simulink model "PathNavShortestRoute"  (R2021a)
settings: Solver=FixedStepDiscrete  StartTime=0.0  StopTime=80  FixedStep=0.01  RelTol=1e-3
values from neighbouring files (symbols this model uses):
  axleLength = 0.136    [robotParameters.m]
  final = makeShort(noZeros)    [createShortPath.m]
  ticksPerRot = 20    [robotParameters.m]
  wheelR = 0.031    [robotParameters.m]
  x = 0.16521    [robotParameters.m]
  y = 0.091117    [robotParameters.m]
undefined symbols (not defined in the file or in its folder): DiscIntNeverNeededParam, InputPWM, lineLength, mapForSim, WheelSpeed
libraries: mobileRoboticsTrainingLib x5, pid_lib x4, simulink_extras x1
settings Model: NumberOfSteps=10  SnapshotBufferSize=100  SnapshotInterval=1  EnablePacing=on  PacingRate=2  Creator=Boitumelo  LastModifiedBy=Marc

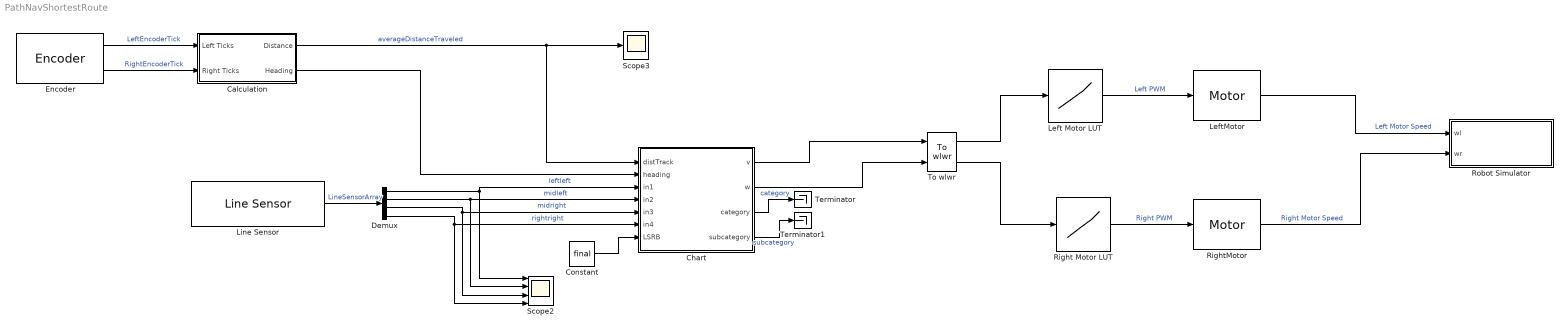
== system PathNavShortestRoute ==
  Calculation : Subsystem
  Chart : Stateflow chart  TreatAsAtomicUnit=on
  Constant : Constant  Value=final
  Demux : Demux
  Encoder : mobileRoboticsTrainingLib/Encoder  axleLength=axleLength  wheelR=wheelR  ticksPerRot=ticksPerRot
      settings: SourceProductName=Mobile Robotics Training Library
  Left Motor LUT : Lookup_n-D  NumberOfTableDimensions=1  BreakpointsForDimension1=WheelSpeed  Table=InputPWM  InterpMethod=Nearest  ExtrapMethod=Clip  InternalRulePriority=Speed  RndMeth=Simplest  InputSameDT=on
  LeftMotor : mobileRoboticsTrainingLib/Motor  motorPlant=wheelMotorModel  sensorType=Speed
      settings: SourceProductName=Mobile Robotics Training Library
  Line Sensor : mobileRoboticsTrainingLib/Line Sensor  mapVariable=mapForSim  envVal=1  lineVal=0  sensOff=[0.0643 0.0354; 0.0675 0.005; 0.0675 -0.005; 0.0643 -0.0354]
      settings: SourceProductName=Mobile Robotics Training Library
  Right Motor LUT : Lookup_n-D  NumberOfTableDimensions=1  BreakpointsForDimension1=WheelSpeed  Table=InputPWM  InterpMethod=Nearest  ExtrapMethod=Clip  InternalRulePriority=Speed  RndMeth=Simplest  InputSameDT=on
  RightMotor : mobileRoboticsTrainingLib/Motor  motorPlant=wheelMotorModel  sensorType=Speed
      settings: SourceProductName=Mobile Robotics Training Library
  Robot Simulator : Subsystem  Priority=99  AncestorBlock=mobileRoboticsTrainingLib/Robot Simulator  mask(Robot Simulator){mapVar=mapForSim, startX=x, startY=y, startTheta=0, axleLength=axleLength, wheelR=wheelR}
      mask prompts: mapVar "Map Variable"; startX "Start X (m)"; startY "Start Y (m)"; startTheta "Theta (deg)"; axleLength "Axle Length (m)"; wheelR "Wheel Radius (m)"
      mask help: Configure robot simulator to use custom simulation maps and simulate closed-loop mobile robotics systems along with appropriate sensor simulation blocks.
      mask init:
      | set_param(bdroot,'SolverType','Fixed-Step');
      | set_param(bdroot,'Solver','FixedStepDiscrete');
      | 
      | if (exist('Ts'))
      |     set_param(bdroot,'FixedStep','Ts');
      | else
      |     set_param(bdroot,'FixedStep','0.01');
      | end
      | 
      | h = findobj('Name','Robot Simulator');
      | if ~isempty(h)
      |     close (h);
      | end
      | setupRobotSim();
      mask Help: web('Robot Simulator.htm')
      mask DialogControl mapCont Prompt: Map Setup
      mask DialogControl initPosCont Prompt: Initial Position
      mask DialogControl setPos Prompt: Set position interactively
      mask DialogControl setPos Callback:
      | %% Set starting point
      | setStartingPoint();
      mask DialogControl initOrientation Prompt: Initial Orientation
      mask DialogControl robotCharCont Prompt: Robot Characteristics
      mask Display: disp('Robot Simulator')
  Scope2 : Scope  NumInputPorts=4
  Scope3 : Scope
  Terminator : Terminator
  Terminator1 : Terminator
  To wlwr : mobileRoboticsTrainingLib/To wlwr  axleLength=0.1  wheelR=0.05
  wires:
  LeftMotor/1 -> Robot Simulator/1(wl)  "Left Motor Speed"
  RightMotor/1 -> Robot Simulator/2(wr)  "Right Motor Speed"
  Right Motor LUT/1 -> RightMotor/1  "Right PWM"
  Left Motor LUT/1 -> LeftMotor/1  "Left PWM"
  To wlwr/1 -> Left Motor LUT/1
  To wlwr/2 -> Right Motor LUT/1
  Line Sensor/1 -> Demux/1  "LineSensorArray"
  Calculation/1(Distance) -> Chart/1(distTrack), Scope3/1  "averageDistanceTraveled"
  Demux/1 -> Scope2/1, Chart/3(in1)  "leftleft"
  Demux/2 -> Scope2/2, Chart/4(in2)  "midleft"
  Demux/3 -> Scope2/3, Chart/5(in3)  "midright"
  Demux/4 -> Scope2/4, Chart/6(in4)  "rightright"
  Chart/1(v) -> To wlwr/1
  Chart/2(w) -> To wlwr/2
  Encoder/1 -> Calculation/1(Left Ticks)  "LeftEncoderTick"
  Encoder/2 -> Calculation/2(Right Ticks)  "RightEncoderTick"
  Calculation/2(Heading) -> Chart/2(heading)
  Chart/3(category) -> Terminator/1  "category"
  Chart/4(subcategory) -> Terminator1/1  "subcategory"
  Constant/1 -> Chart/7(LSRB)

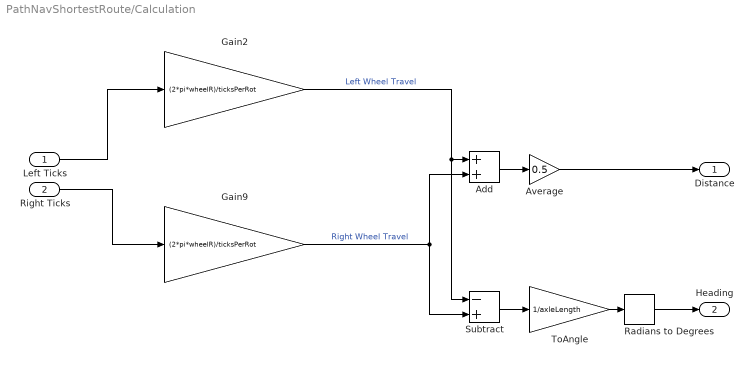
== system PathNavShortestRoute/Calculation ==
  Left Ticks : Inport
  Right Ticks : Inport  Port=2
  Add : Sum
  Average : Gain  Gain=0.5
  Gain2 : Gain  Gain=(2*pi*wheelR)/ticksPerRot
  Gain9 : Gain  Gain=(2*pi*wheelR)/ticksPerRot
  Radians to Degrees : simulink_extras/Transformations/Radians to Degrees
  Subtract : Sum  Inputs=-+
  ToAngle : Gain  Gain=1/axleLength
  Distance : Outport
  Heading : Outport  Port=2
  wires:
  Average/1 -> Distance/1
  Add/1 -> Average/1
  Gain2/1 -> Subtract/1, Add/1  "Left Wheel Travel"
  Right Ticks/1 -> Gain9/1
  Left Ticks/1 -> Gain2/1
  Gain9/1 -> Subtract/2, Add/2  "Right Wheel Travel"
  Subtract/1 -> ToAngle/1
  ToAngle/1 -> Radians to Degrees/1
  Radians to Degrees/1 -> Heading/1

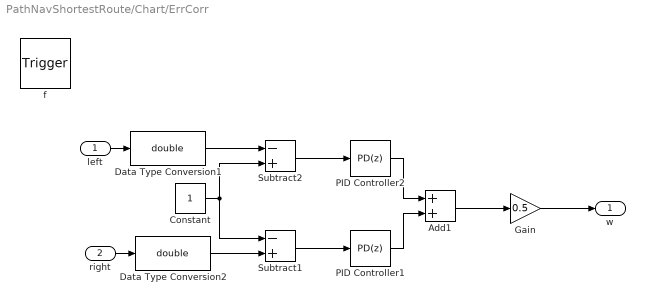
== system PathNavShortestRoute/Chart/ErrCorr ==
  left : Inport  OutDataTypeStr=double  PortDimensions=1
  right : Inport  Port=2  OutDataTypeStr=double  PortDimensions=1
  f : TriggerPort  TriggerType=function-call  VariantControl=(inherit)
      settings: CopyFcn=Stateflow.SLINSF.SimulinkMan.removeBlockPreDeleteFcn  PreDeleteFcn=Stateflow.SLINSF.SimulinkMan.unsafePredeleteFcn
  Add1 : Sum
  Constant : Constant
  Data Type Conversion1 : DataTypeConversion  OutDataTypeStr=double
  Data Type Conversion2 : DataTypeConversion  OutDataTypeStr=double
  Gain : Gain  Gain=0.5
  PID Controller1 : pid_lib/PID Controller  Controller=PD  Form=Parallel  TimeDomain=Discrete-time  UseExternalTs=off  SampleTime=-1  IntegratorMethod=Forward Euler  FilterMethod=Forward Euler  ControllerParametersSource=internal  P=1.5  I=1  D=1e-5  UseFilter=on  N=100  TunerSelectOption=Transfer Function Based (PID Tuner App)  InitialConditionSource=internal  InitialConditionForIntegrator=0  InitialConditionForFilter=0  DifferentiatorICPrevScaledInput=0  ExternalReset=none  TrackingMode=off  Kt=1  LimitOutput=off  SatLimitsSource=internal  UpperSaturationLimit=inf  LowerSaturationLimit=-inf  LinearizeAsGain=on  AntiWindupMode=none  Kb=1  POutMin=[]  POutMax=[]  IOutMin=[]  IOutMax=[]  DOutMin=[]  DOutMax=[]  NOutMin=[]  NOutMax=[]  SumOutMin=[]  SumOutMax=[]  SaturationOutMin=[]  SaturationOutMax=[]  PParamMin=[]  PParamMax=[]  IParamMin=[]  IParamMax=[]  DParamMin=[]  DParamMax=[]  NParamMin=[]  NParamMax=[]  KbParamMin=[]  KbParamMax=[]  KtParamMin=[]  KtParamMax=[]  KbOutMin=[]  KbOutMax=[]  KtOutMin=[]  KtOutMax=[]  IntegratorOutMin=[]  IntegratorOutMax=[]  FilterOutMin=[]  FilterOutMax=[]  SumI1OutMin=[]  SumI1OutMax=[]  SumI2OutMin=[]  SumI2OutMax=[]  SumI3OutMin=[]  SumI3OutMax=[]  SumI4OutMin=[]  SumI4OutMax=[]  SumDOutMin=[]  SumDOutMax=[]  DifferentiatorOutMin=[]  DifferentiatorOutMax=[]  FilterDiffOutCoefMin=[]  FilterDiffOutCoefMax=[]  ReciprocalOutMin=[]  ReciprocalOutMax=[]  SumDenOutMin=[]  SumDenOutMax=[]  SumNumOutMin=[]  SumNumOutMax=[]  DivideOutMin=[]  DivideOutMax=[]  UdiffTsProdOutMin=[]  UdiffTsProdOutMax=[]  NTsProdOutMin=[]  NTsProdOutMax=[]  UintegralTsProdOutMin=[]  UintegralTsProdOutMax=[]  UngainTsProdOutMin=[]  UngainTsProdOutMax=[]  IntegratorContinuousStateAttributes=''  IntegratorStateMustResolveToSignalObject=off  IntegratorRTWStateStorageClass=Auto  FilterContinuousStateAttributes=''  FilterStateMustResolveToSignalObject=off  FilterRTWStateStorageClass=Auto  ParallelPVariant=InternalParameters  IdealPVariant=Disabled  IVariant=Disabled  DVariant=InternalParameters  IntegratorVariant=Disabled  SatVariant=Disabled  AWVariant=Disabled  PCopyVariant=Disabled  TRVariant=Disabled  FdbkBlocksVariant=Forward  IdealPFdbkVariant=Disabled  SatFdbkVariant=Disabled  DerivativeFilterVariant=ForwardEulerFilter  NVariant=InternalParameters  NCopyVariant=Disabled  FilterICVariant=InternalICsFilter  IntegratorICVariant=Disabled  ExternalResetVariant=Disabled  TRSumVariant=Passthrough  SumFdbkVariant=Disabled  SumVariant=Sum_PD  TsampFilterVariant=InternalTs  TsampNgainVariant=Passthrough  TsampIntegralVariant=Disabled_SignalSpec  ExternalSaturationOutDataTypeStr=Inherit: Same as second input  InitialConditionSetting=Output
  PID Controller2 : pid_lib/PID Controller  Controller=PD  Form=Parallel  TimeDomain=Discrete-time  UseExternalTs=off  SampleTime=-1  IntegratorMethod=Forward Euler  FilterMethod=Forward Euler  ControllerParametersSource=internal  P=1.5  I=1  D=1e-5  UseFilter=on  N=100  TunerSelectOption=Transfer Function Based (PID Tuner App)  InitialConditionSource=internal  InitialConditionForIntegrator=0  InitialConditionForFilter=0  DifferentiatorICPrevScaledInput=0  ExternalReset=none  TrackingMode=off  Kt=1  LimitOutput=off  SatLimitsSource=internal  UpperSaturationLimit=inf  LowerSaturationLimit=-inf  LinearizeAsGain=on  AntiWindupMode=none  Kb=1  POutMin=[]  POutMax=[]  IOutMin=[]  IOutMax=[]  DOutMin=[]  DOutMax=[]  NOutMin=[]  NOutMax=[]  SumOutMin=[]  SumOutMax=[]  SaturationOutMin=[]  SaturationOutMax=[]  PParamMin=[]  PParamMax=[]  IParamMin=[]  IParamMax=[]  DParamMin=[]  DParamMax=[]  NParamMin=[]  NParamMax=[]  KbParamMin=[]  KbParamMax=[]  KtParamMin=[]  KtParamMax=[]  KbOutMin=[]  KbOutMax=[]  KtOutMin=[]  KtOutMax=[]  IntegratorOutMin=[]  IntegratorOutMax=[]  FilterOutMin=[]  FilterOutMax=[]  SumI1OutMin=[]  SumI1OutMax=[]  SumI2OutMin=[]  SumI2OutMax=[]  SumI3OutMin=[]  SumI3OutMax=[]  SumI4OutMin=[]  SumI4OutMax=[]  SumDOutMin=[]  SumDOutMax=[]  DifferentiatorOutMin=[]  DifferentiatorOutMax=[]  FilterDiffOutCoefMin=[]  FilterDiffOutCoefMax=[]  ReciprocalOutMin=[]  ReciprocalOutMax=[]  SumDenOutMin=[]  SumDenOutMax=[]  SumNumOutMin=[]  SumNumOutMax=[]  DivideOutMin=[]  DivideOutMax=[]  UdiffTsProdOutMin=[]  UdiffTsProdOutMax=[]  NTsProdOutMin=[]  NTsProdOutMax=[]  UintegralTsProdOutMin=[]  UintegralTsProdOutMax=[]  UngainTsProdOutMin=[]  UngainTsProdOutMax=[]  IntegratorContinuousStateAttributes=''  IntegratorStateMustResolveToSignalObject=off  IntegratorRTWStateStorageClass=Auto  FilterContinuousStateAttributes=''  FilterStateMustResolveToSignalObject=off  FilterRTWStateStorageClass=Auto  ParallelPVariant=InternalParameters  IdealPVariant=Disabled  IVariant=Disabled  DVariant=InternalParameters  IntegratorVariant=Disabled  SatVariant=Disabled  AWVariant=Disabled  PCopyVariant=Disabled  TRVariant=Disabled  FdbkBlocksVariant=Forward  IdealPFdbkVariant=Disabled  SatFdbkVariant=Disabled  DerivativeFilterVariant=ForwardEulerFilter  NVariant=InternalParameters  NCopyVariant=Disabled  FilterICVariant=InternalICsFilter  IntegratorICVariant=Disabled  ExternalResetVariant=Disabled  TRSumVariant=Passthrough  SumFdbkVariant=Disabled  SumVariant=Sum_PD  TsampFilterVariant=InternalTs  TsampNgainVariant=Passthrough  TsampIntegralVariant=Disabled_SignalSpec  ExternalSaturationOutDataTypeStr=Inherit: Same as second input  InitialConditionSetting=Output
  Subtract1 : Sum  Inputs=-+
  Subtract2 : Sum  Inputs=-+
  w : Outport
  wires:
  Subtract2/1 -> PID Controller2/1
  Subtract1/1 -> PID Controller1/1
  PID Controller1/1 -> Add1/2
  Constant/1 -> Subtract2/2, Subtract1/1
  left/1 -> Data Type Conversion1/1
  right/1 -> Data Type Conversion2/1
  PID Controller2/1 -> Add1/1
  Add1/1 -> Gain/1
  Data Type Conversion2/1 -> Subtract1/2
  Data Type Conversion1/1 -> Subtract2/1
  Gain/1 -> w/1

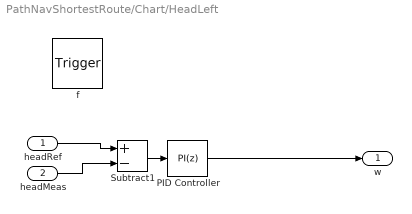
== system PathNavShortestRoute/Chart/HeadLeft ==
  headRef : Inport  OutDataTypeStr=double  PortDimensions=1
  headMeas : Inport  Port=2  OutDataTypeStr=double  PortDimensions=1
  f : TriggerPort  TriggerType=function-call  VariantControl=(inherit)
      settings: CopyFcn=Stateflow.SLINSF.SimulinkMan.removeBlockPreDeleteFcn  PreDeleteFcn=Stateflow.SLINSF.SimulinkMan.unsafePredeleteFcn
  PID Controller : pid_lib/PID Controller  Controller=PI  Form=Parallel  TimeDomain=Discrete-time  UseExternalTs=off  SampleTime=-1  IntegratorMethod=Forward Euler  FilterMethod=Forward Euler  ControllerParametersSource=internal  P=0.1  I=0.001  D=-0.0140783779685636  UseFilter=off  N=151.701833251505  TunerSelectOption=Transfer Function Based (PID Tuner App)  InitialConditionSource=internal  InitialConditionForIntegrator=0  InitialConditionForFilter=0  DifferentiatorICPrevScaledInput=0  ExternalReset=none  TrackingMode=off  Kt=1  LimitOutput=on  SatLimitsSource=internal  UpperSaturationLimit=4  LowerSaturationLimit=-4  LinearizeAsGain=on  AntiWindupMode=clamping  Kb=1  POutMin=[]  POutMax=[]  IOutMin=[]  IOutMax=[]  DOutMin=[]  DOutMax=[]  NOutMin=[]  NOutMax=[]  SumOutMin=[]  SumOutMax=[]  SaturationOutMin=[]  SaturationOutMax=[]  PParamMin=[]  PParamMax=[]  IParamMin=[]  IParamMax=[]  DParamMin=[]  DParamMax=[]  NParamMin=[]  NParamMax=[]  KbParamMin=[]  KbParamMax=[]  KtParamMin=[]  KtParamMax=[]  KbOutMin=[]  KbOutMax=[]  KtOutMin=[]  KtOutMax=[]  IntegratorOutMin=[]  IntegratorOutMax=[]  FilterOutMin=[]  FilterOutMax=[]  SumI1OutMin=[]  SumI1OutMax=[]  SumI2OutMin=[]  SumI2OutMax=[]  SumI3OutMin=[]  SumI3OutMax=[]  SumI4OutMin=[]  SumI4OutMax=[]  SumDOutMin=[]  SumDOutMax=[]  DifferentiatorOutMin=[]  DifferentiatorOutMax=[]  FilterDiffOutCoefMin=[]  FilterDiffOutCoefMax=[]  ReciprocalOutMin=[]  ReciprocalOutMax=[]  SumDenOutMin=[]  SumDenOutMax=[]  SumNumOutMin=[]  SumNumOutMax=[]  DivideOutMin=[]  DivideOutMax=[]  UdiffTsProdOutMin=[]  UdiffTsProdOutMax=[]  NTsProdOutMin=[]  NTsProdOutMax=[]  UintegralTsProdOutMin=[]  UintegralTsProdOutMax=[]  UngainTsProdOutMin=[]  UngainTsProdOutMax=[]  IntegratorContinuousStateAttributes=''  IntegratorStateMustResolveToSignalObject=off  IntegratorRTWStateStorageClass=Auto  FilterContinuousStateAttributes=''  FilterStateMustResolveToSignalObject=off  FilterRTWStateStorageClass=Auto  ParallelPVariant=InternalParameters  IdealPVariant=Disabled  IVariant=InternalParameters  DVariant=Disabled  IntegratorVariant=Discrete  SatVariant=Enabled  AWVariant=DiscClampingParallel  PCopyVariant=Disabled  TRVariant=Disabled  FdbkBlocksVariant=Forward  IdealPFdbkVariant=Disabled  SatFdbkVariant=Disabled  DerivativeFilterVariant=Disabled  NVariant=Disabled  NCopyVariant=Disabled_SignalSpec  FilterICVariant=Disabled  IntegratorICVariant=InternalICs  ExternalResetVariant=Disabled  TRSumVariant=Passthrough  SumFdbkVariant=Disabled  SumVariant=Sum_PI  TsampFilterVariant=InternalTs  TsampNgainVariant=Passthrough  TsampIntegralVariant=Passthrough  ExternalSaturationOutDataTypeStr=Inherit: Same as second input  InitialConditionSetting=Output
  Subtract1 : Sum  Inputs=+-
  w : Outport
  wires:
  Subtract1/1 -> PID Controller/1
  headMeas/1 -> Subtract1/2
  headRef/1 -> Subtract1/1
  PID Controller/1 -> w/1

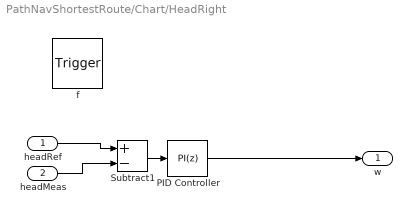
== system PathNavShortestRoute/Chart/HeadRight ==
  headRef : Inport  OutDataTypeStr=double  PortDimensions=1
  headMeas : Inport  Port=2  OutDataTypeStr=double  PortDimensions=1
  f : TriggerPort  TriggerType=function-call  VariantControl=(inherit)
      settings: CopyFcn=Stateflow.SLINSF.SimulinkMan.removeBlockPreDeleteFcn  PreDeleteFcn=Stateflow.SLINSF.SimulinkMan.unsafePredeleteFcn
  PID Controller : pid_lib/PID Controller  Controller=PI  Form=Parallel  TimeDomain=Discrete-time  UseExternalTs=off  SampleTime=-1  IntegratorMethod=Forward Euler  FilterMethod=Forward Euler  ControllerParametersSource=internal  P=0.1  I=0.001  D=-0.0140783779685636  UseFilter=off  N=151.701833251505  TunerSelectOption=Transfer Function Based (PID Tuner App)  InitialConditionSource=internal  InitialConditionForIntegrator=0  InitialConditionForFilter=0  DifferentiatorICPrevScaledInput=0  ExternalReset=none  TrackingMode=off  Kt=1  LimitOutput=on  SatLimitsSource=internal  UpperSaturationLimit=4  LowerSaturationLimit=-4  LinearizeAsGain=on  AntiWindupMode=clamping  Kb=1  POutMin=[]  POutMax=[]  IOutMin=[]  IOutMax=[]  DOutMin=[]  DOutMax=[]  NOutMin=[]  NOutMax=[]  SumOutMin=[]  SumOutMax=[]  SaturationOutMin=[]  SaturationOutMax=[]  PParamMin=[]  PParamMax=[]  IParamMin=[]  IParamMax=[]  DParamMin=[]  DParamMax=[]  NParamMin=[]  NParamMax=[]  KbParamMin=[]  KbParamMax=[]  KtParamMin=[]  KtParamMax=[]  KbOutMin=[]  KbOutMax=[]  KtOutMin=[]  KtOutMax=[]  IntegratorOutMin=[]  IntegratorOutMax=[]  FilterOutMin=[]  FilterOutMax=[]  SumI1OutMin=[]  SumI1OutMax=[]  SumI2OutMin=[]  SumI2OutMax=[]  SumI3OutMin=[]  SumI3OutMax=[]  SumI4OutMin=[]  SumI4OutMax=[]  SumDOutMin=[]  SumDOutMax=[]  DifferentiatorOutMin=[]  DifferentiatorOutMax=[]  FilterDiffOutCoefMin=[]  FilterDiffOutCoefMax=[]  ReciprocalOutMin=[]  ReciprocalOutMax=[]  SumDenOutMin=[]  SumDenOutMax=[]  SumNumOutMin=[]  SumNumOutMax=[]  DivideOutMin=[]  DivideOutMax=[]  UdiffTsProdOutMin=[]  UdiffTsProdOutMax=[]  NTsProdOutMin=[]  NTsProdOutMax=[]  UintegralTsProdOutMin=[]  UintegralTsProdOutMax=[]  UngainTsProdOutMin=[]  UngainTsProdOutMax=[]  IntegratorContinuousStateAttributes=''  IntegratorStateMustResolveToSignalObject=off  IntegratorRTWStateStorageClass=Auto  FilterContinuousStateAttributes=''  FilterStateMustResolveToSignalObject=off  FilterRTWStateStorageClass=Auto  ParallelPVariant=InternalParameters  IdealPVariant=Disabled  IVariant=InternalParameters  DVariant=Disabled  IntegratorVariant=Discrete  SatVariant=Enabled  AWVariant=DiscClampingParallel  PCopyVariant=Disabled  TRVariant=Disabled  FdbkBlocksVariant=Forward  IdealPFdbkVariant=Disabled  SatFdbkVariant=Disabled  DerivativeFilterVariant=Disabled  NVariant=Disabled  NCopyVariant=Disabled_SignalSpec  FilterICVariant=Disabled  IntegratorICVariant=InternalICs  ExternalResetVariant=Disabled  TRSumVariant=Passthrough  SumFdbkVariant=Disabled  SumVariant=Sum_PI  TsampFilterVariant=InternalTs  TsampNgainVariant=Passthrough  TsampIntegralVariant=Passthrough  ExternalSaturationOutDataTypeStr=Inherit: Same as second input  InitialConditionSetting=Output
  Subtract1 : Sum  Inputs=+-
  w : Outport
  wires:
  Subtract1/1 -> PID Controller/1
  headMeas/1 -> Subtract1/2
  headRef/1 -> Subtract1/1
  PID Controller/1 -> w/1

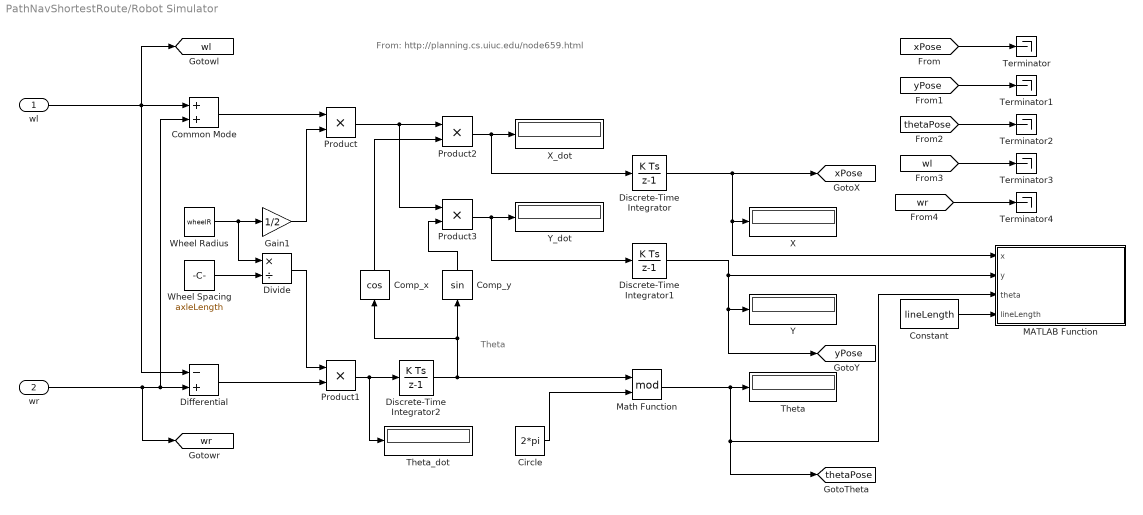
== system PathNavShortestRoute/Robot Simulator ==
  note: Theta
  note: From: http://planning.cs.uiuc.edu/node659.html
  wl : Inport
  wr : Inport  Port=2
  Circle : Constant  Value=2*pi
  Common Mode : Sum
  Comp_x : Trigonometry  Operator=cos
  Comp_y : Trigonometry
  Constant : Constant  Value=lineLength
  Differential : Sum  Inputs=-+
  Discrete-Time Integrator : DiscreteIntegrator  InitialCondition=startX  SampleTime=-1  ICPrevOutput=DiscIntNeverNeededParam  ICPrevScaledInput=DiscIntNeverNeededParam
  Discrete-Time Integrator1 : DiscreteIntegrator  InitialCondition=startY  SampleTime=-1  ICPrevOutput=DiscIntNeverNeededParam  ICPrevScaledInput=DiscIntNeverNeededParam
  Discrete-Time Integrator2 : DiscreteIntegrator  InitialCondition=startTheta*(pi/180)  SampleTime=-1  ICPrevOutput=DiscIntNeverNeededParam  ICPrevScaledInput=DiscIntNeverNeededParam
  Divide : Product  Inputs=*/
  Gain1 : Gain  Gain=1/2
  MATLAB Function : MATLAB Function  TreatAsAtomicUnit=on
  Math Function : Math  Operator=mod  SignedPower=on  SaturateOnIntegerOverflow=on
  Product{,1..3} (4 alike) : Product  RndMeth=Zero
  Terminator{,1..4} (5 alike) : Terminator
  Theta : Display
  Theta_dot : Display
  Wheel Radius : Constant  Value=wheelR
  Wheel Spacing : Constant  Value=axleLength
  X : Display
  X_dot : Display
  Y : Display
  Y_dot : Display
  tag scope: thetaPose=global, wl=global, wr=global, xPose=global, yPose=global
  wires:
  [wr] -> Terminator4/1
  [wl] -> Terminator3/1
  Math Function/1 -> [thetaPose], MATLAB Function/3(theta), Theta/1
  Differential/1 -> Product1/2
  Comp_y/1 -> Product3/2
  Discrete-Time Integrator/1 -> [xPose], MATLAB Function/1(x), X/1
  Product3/1 -> Discrete-Time Integrator1/1, Y_dot/1
  Discrete-Time Integrator1/1 -> Y/1, [yPose], MATLAB Function/2(y)
  Divide/1 -> Product1/1
  wr/1 -> [wr], Common Mode/2, Differential/2
  Discrete-Time Integrator2/1 -> Math Function/1, Comp_x/1, Comp_y/1
  wl/1 -> [wl], Common Mode/1, Differential/1
  Comp_x/1 -> Product2/2
  Product1/1 -> Discrete-Time Integrator2/1, Theta_dot/1
  Wheel Radius/1 -> Divide/1, Gain1/1
  Wheel Spacing/1 -> Divide/2
  Product2/1 -> Discrete-Time Integrator/1, X_dot/1
  Gain1/1 -> Product/2
  Common Mode/1 -> Product/1
  Product/1 -> Product3/1, Product2/1
  Circle/1 -> Math Function/2
  Constant/1 -> MATLAB Function/4(lineLength)
  [xPose] -> Terminator/1
  [yPose] -> Terminator1/1
  [thetaPose] -> Terminator2/1

== matlab function PathNavShortestRoute/Robot Simulator/MATLAB Function ==
  data: x input; y input; theta input; lineLength input
function plotRobot(x,y,theta,lineLength)
% Get plot details
coder.extrinsic('evalin','plot')
ph1 = evalin('base','PlotHandle1');
ph2 = evalin('base','PlotHandle2');

% Find length orientation line
xp = [x x+lineLength*cos(theta)];
yp = [y y+lineLength*sin(theta)];

% Plot robot
set(ph1,'xdata',xp,'ydata',yp);
set(ph2,'xdata',x,'ydata',y);
drawnow('limitrate')

== stateflow chart PathNavShortestRoute/Chart ==
  state w=HeadLeft(headRef,headMeas) [function]
  state w=ErrCorr(left,right) [function]
  state w=HeadRight(headRef,headMeas) [function]
  state Initial
    entry:
    n=1;
  state LineFollow
    state EndOfMaze
      entry:
      v=0;
      w=0;
      subcategory= 1;
    state TurnLeft
      entry:
      w= 4
      exit:
      w=0
    state TurnRight
      entry:
      w= -4
      exit:
      w=0
    state CrossRoads
      entry:
      v=0;
      w=0;
      subcategory= 2;
    state Junction1_0000_
      entry:
      v=0.1;
      w=0;
      stopDist=0.018
      startDist = distTrack
      category = 2
    state MoveForward
      entry:
      v=0.2;
      stopDist=2
      category = 1
      %during:
      %w=ErrCorr(in2,in3);
    state J0000
      entry:
      v=0
    state TJunc
      entry:
      v=0;
      w=0;
      subcategory= 3;
    state Initial
      entry:
      v=0;
      w=0;
      stopDist=0;
      category= 0;
    state StartDetect
      entry,during:
      stopDist=0
      %v=0.05
      w=ErrCorr(in2,in3);
    state Junction2_1000_
      entry:
      v=0.1;
      w=0;
      stopDist=0.018
      startDist = distTrack
      category = 3
    state RightTurn
      entry:
      v=0;
      w=0;
      subcategory= 1;
    state J1000
      entry:
      v=0
      during:
      % w=ErrCorr(in2,in3)
    state JunctionDetected
      entry:
      x=LSRB(n)
    state RightTJunc
      entry:
      v=0;
      w=0;
      subcategory= 2;
    state Junction3_0001_
      entry:
      v=0.1;
      w=0;
      stopDist=0.018
      startDist = distTrack
      category = 4
    state J0001
      entry:
      v=0
    state LeftTurn
      entry:
      v=0;
      w=0;
      subcategory= 1;
    state DeadEnd1
    state LeftTJunc
      entry:
      v=0;
      w=0;
      subcategory= 2;
    state DeadEnd
      entry:
      v=0;
      w=0;
      category = 5
      subcategory= 1;
    Junction1_0000_ -> EndOfMaze [order 1] : [distTrack >= (startDist + 0.075) & in1==0 & in2==0 & in3==0 & in4==0 ]
    MoveForward -> TurnLeft [order 1] : [in2==0 & in3==1]
    TurnLeft -> MoveForward : [in2==0 & in3==0]
    MoveForward -> TurnRight [order 2] : [in2==1 & in3==0]
    TurnRight -> MoveForward : [in2==0 & in3==0]
    CrossRoads -> JunctionDetected
    Junction1_0000_ -> CrossRoads [order 2] : [distTrack >= (startDist +0.059) & in1==1 & in2==0 & in3==0 & in4==1 ]
    (default) -> LineFollow.Initial
    MoveForward -> J0000 [order 3] : [in1==0 & in2==0 & in3==0 & in4==0]
    Junction1_0000_ -> TJunc [order 3] : [distTrack >= (startDist + 0.059) & in1==1 & in2==1 & in3==1 & in4==1 ]
    J0000 -> MoveForward [order 2] : [in1==1 || in4==1]
    J0000 -> Junction1_0000_ [order 1] : after(0.01,sec) [in1==0 & in2==0 & in3==0 & in4==0]
    StartDetect -> MoveForward : [in2==0 & in3==0]
    LineFollow.Initial -> StartDetect
    TJunc -> JunctionDetected
    Junction2_1000_ -> RightTurn [order 1] : [distTrack >= (startDist + 0.059) & in1==1 & in2==1 & in3==1 & in4==1 ]
    MoveForward -> J1000 [order 4] : [in1==1 & in2==0 & in3==0 & in4==0]
    RightTurn -> JunctionDetected
    Junction2_1000_ -> RightTJunc [order 2] : [distTrack >= (startDist + 0.059) & in1==1 & in2==0 & in3==0 & in4==1 ]
    J1000 -> MoveForward [order 2] : [in1==0 || in4==1]
    J1000 -> Junction2_1000_ [order 1] : after(0.1,sec) [in1==1 & in2==0 & in3==0 & in4==0]
    RightTJunc -> JunctionDetected
    DeadEnd1 -> MoveForward [order 1] : [in1==0 || in2==0 || in3==0 || in4==0]
    MoveForward -> DeadEnd1 [order 6] : [in1==1 & in2==1 & in3==1 & in4==1]
    J0001 -> MoveForward [order 2] : [in1==1 || in4==0]
    MoveForward -> J0001 [order 5] : [in1==0 & in2==0 & in3==0 & in4==1]
    LeftTJunc -> JunctionDetected
    LeftTurn -> JunctionDetected
    DeadEnd -> JunctionDetected
    J0001 -> Junction3_0001_ [order 1] : after(0.01, sec) [in1==0 & in2==0 & in3==0 & in4==1]
    Junction3_0001_ -> LeftTurn [order 1] : [distTrack >= (startDist + 0.059) & in1==1 & in2==1 & in3==1 & in4==1]
    Junction3_0001_ -> LeftTJunc [order 2] : [distTrack >= (startDist + 0.059) & in1==1 & in2==0 & in3==0 & in4==1 ]
    DeadEnd1 -> DeadEnd [order 2] : after(0.05,sec) [in1==1 & in2==1 & in3==1 & in4==1]
  state Left
    state Rotate
      entry:
      currHead=heading
      n=n+1;
      during:
      w=HeadLeft(90+currHead,heading);
      %doing=1;
    state Stop
      entry:
      w=0
      currHead=heading
      doing=0;
    (default) -> Left.Rotate
    Left.Rotate -> Left.Stop : [heading-currHead>=90]{currHead=heading}
  state Straight
    state Initial
      entry:
      n=n+1;
      doing=1;
    state End
      entry:
      doing=0;
    (default) -> Straight.Initial
    Straight.Initial -> End
  state Right
    state Rotate
      entry:
      currHead=heading
      doing=1;
      n=n+1;
      during:
      w=HeadRight(currHead-90,heading);
    state Stop
      entry:
      w=0
      doing=0;
      currHead=heading
    (default) -> Right.Rotate
    Right.Rotate -> Right.Stop : [heading-currHead<=-90]{currHead=heading}
  state Back
    state Rotate
      entry:
      currHead=heading
      doing=1;
      n=n+1;
      during:
      w=HeadLeft(180+currHead,heading);
    state Stop
      entry:
      w=0
      doing=0;
    (default) -> Back.Rotate
    Back.Rotate -> Back.Stop : [heading-currHead>=180]{currHead=heading}
  (default) -> Initial
  Initial -> LineFollow
  JunctionDetected -> Left [order 1] : [x==1]
  Left.Stop -> LineFollow : after(0.25,sec)
  JunctionDetected -> Straight [order 3] : [x==2]
  End -> LineFollow
  JunctionDetected -> Right [order 4] : [x==3]
  JunctionDetected -> Back [order 2] : [x==4]
  Right.Stop -> LineFollow : after(0.25,sec)
  Back -> LineFollow : after(0.25,sec)
  data: headRef function_input double size=1; headMeas function_input double size=1; w function_output; left function_input double size=1; right function_input double size=1; w function_output; headRef function_input double size=1; headMeas function_input double size=1; w function_output; distTrack input; heading input; in1 input; in2 input; in3 input; in4 input; v output; w output; category output; subcategory output; startDist local; stopDist local; currHead local; LSRB input; doing local; x local; n local
